simulink model "test"  (R2014b)
settings: Solver=ode45  StartTime=0.0  StopTime=10.0  RelTol=1e-3
undefined symbols (not defined in the file or in its folder): i
settings Model: Creator=kjartan  LastModifiedBy=kjartan

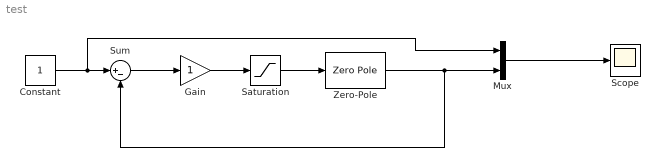
== system test ==
  Constant : Constant
  Gain : Gain
  Mux : Mux  Inputs=2
  Saturation : Saturate
  Scope : Scope
  Sum : Sum  Inputs=|+-
  Zero-Pole : ZeroPole  Zeros=[-3]  Poles=[0 -2 -1+2*i -1-2*i]  Gain=[5]
  wires:
  Zero-Pole/1 -> Sum/2, Mux/2
  Mux/1 -> Scope/1
  Sum/1 -> Gain/1
  Gain/1 -> Saturation/1
  Saturation/1 -> Zero-Pole/1
  Constant/1 -> Mux/1, Sum/1
